simulink model "CoolingLoopModel"  (R2025b)
settings: Solver=VariableStepAuto  StartTime=0.0  StopTime=3600  RelTol=1e-3
values from neighbouring files (symbols this model uses):
  Cp = 3500    [setup_cooling_loop.m]
  Flow_Rate = 0.2    [setup_cooling_loop.m]
  Mass = rho * Vol    (= 5.3)    [setup_cooling_loop.m]
  T_ambient = 25    [setup_cooling_loop.m]
  T_init = 25    [setup_cooling_loop.m]
  UA_rated = 150    [setup_cooling_loop.m]

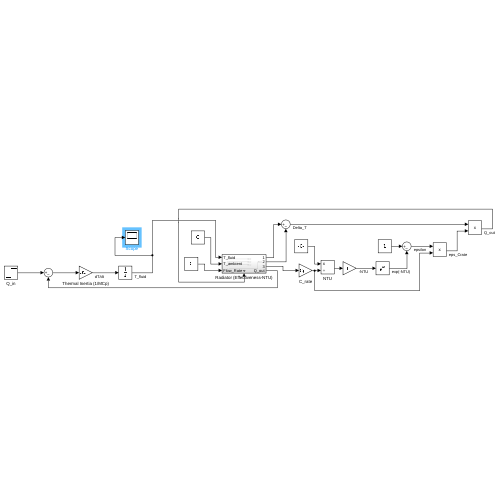
[thumbnail: Simulink's stored preview of the top-level diagram]
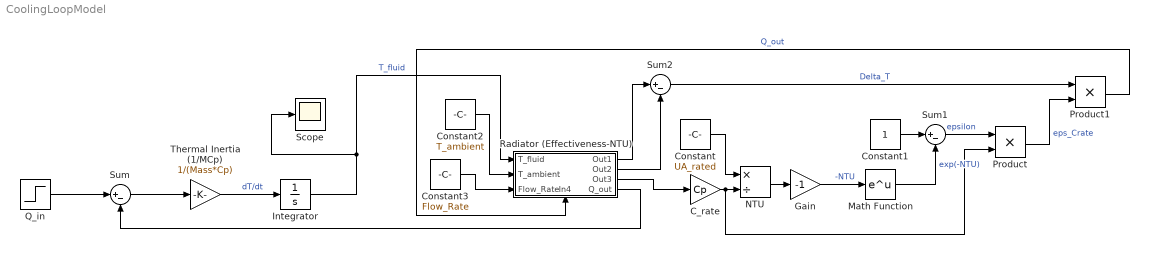
== system CoolingLoopModel ==
  C_rate : Gain  Gain=Cp
  Constant : Constant  Value=UA_rated
  Constant1 : Constant
  Constant2 : Constant  Value=T_ambient
  Constant3 : Constant  Value=Flow_Rate
  Gain : Gain  Gain=-1
  Integrator : Integrator  InitialCondition=T_init
  Math Function : Math
  NTU : Product  Inputs=*/
  Product : Product
  Product1 : Product
  Q_in : Step  Time=10  After=1000  SampleTime=0
  Radiator (Effectiveness-NTU) : Subsystem
      settings: PortSchema="{\"entries\":[{\"content\":{\"sides\":[{\"content\":{\"connectorIds\":[\"In1\",\"In2\",\"In3\"]},\"type\":\"ConnectorPlacement.EquallySpacedRectSide\",\"uuid\":\"763b49ba-e30a-4bf7-9101-0a483e23a5d2\"},{\"content\":{\"connectorIds\":[\"Out1\",\"Out2\",\"Out3\",\"Out4\"],\"side\":\"RIGHT\"},\"type\":\"ConnectorPlacement.EquallySpacedRectSide\",\"uuid\":\"15db3555-d9f1-4d5e-8554-55ba6d53e958\"},{\"content\":{\"side\":\"TOP\"},\"type\":\"ConnectorPlacement.EquallySpacedRectSide\",\"uuid\":\"2fa32cb6-28f3-4e76-9763-bb31515744bd\"},{\"content\":{\"connectorIds\":[\"In4\"],\"side\":\"BOTTOM\"},\"type\":\"ConnectorPlacement.EquallySpacedRectSide\",\"uuid\":\"8386595c-2f4c-4c89-910d-26e6f3067b4d\"}]},\"type\":\"ConnectorPlacement.EquallySpacedConnector\",\"uuid\":\"c16c71c5-6ab8-4f10-96ea-2b59fe03dc5f\"}],\"packageUris\":[\"http://schema.mathworks.com/mf0/Connector/R2020b\"],\"version\":\"1.0\"}"
  Scope : Scope
      settings: ActiveDisplayYMinimum=24.074194614599321  ActiveDisplayYMaximum=33.332248468606117
  Sum : Sum  Inputs=|+-
  Sum1 : Sum  Inputs=|+-
  Sum2 : Sum  Inputs=|+-
  Thermal Inertia (1/MCp) : Gain  Gain=1/(Mass*Cp)
  wires:
  Q_in/1 -> Sum/1
  Sum/1 -> Thermal Inertia (1/MCp)/1
  Thermal Inertia (1/MCp)/1 -> Integrator/1  "dT/dt"
  Radiator (Effectiveness-NTU)/3(Out3) -> C_rate/1
  C_rate/1 -> Product/2, NTU/2
  Constant/1 -> NTU/1
  NTU/1 -> Gain/1
  Gain/1 -> Math Function/1  "-NTU"
  Constant1/1 -> Sum1/1
  Math Function/1 -> Sum1/2  "exp(-NTU)"
  Radiator (Effectiveness-NTU)/1(Out1) -> Sum2/1
  Radiator (Effectiveness-NTU)/2(Out2) -> Sum2/2
  Sum1/1 -> Product/1  "epsilon"
  Product/1 -> Product1/2  "eps_Crate"
  Sum2/1 -> Product1/1  "Delta_T"
  Product1/1 -> Radiator (Effectiveness-NTU)/4(In4)  "Q_out"
  Radiator (Effectiveness-NTU)/4(Q_out) -> Sum/2
  Integrator/1 -> Radiator (Effectiveness-NTU)/1(T_fluid), Scope/1  "T_fluid"
  Constant2/1 -> Radiator (Effectiveness-NTU)/2(T_ambient)
  Constant3/1 -> Radiator (Effectiveness-NTU)/3(Flow_Rate)

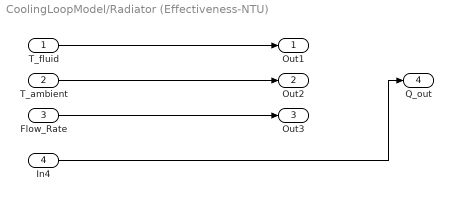
== system CoolingLoopModel/Radiator (Effectiveness-NTU) ==
  T_fluid : Inport
  T_ambient : Inport  Port=2
  Flow_Rate : Inport  Port=3
  In4 : Inport  Port=4
  Out1 : Outport
  Out2 : Outport  Port=2
  Out3 : Outport  Port=3
  Q_out : Outport  Port=4
  wires:
  T_fluid/1 -> Out1/1
  T_ambient/1 -> Out2/1
  Flow_Rate/1 -> Out3/1
  In4/1 -> Q_out/1
